simulink model "plots"  (R2014b)
settings: Solver=FixedStepDiscrete  StartTime=0.0  StopTime=inf  FixedStep=Ts  RelTol=1e-3
InitFcn:
  | Ts=0.010;
  | ROBOT_DOF=23;
  | robotName='icubGazeboSim';
  | localName='simulink';
libraries: WBCLibrary x2
settings Model: Creator=jorhabib  LastModifiedBy=jorhabib

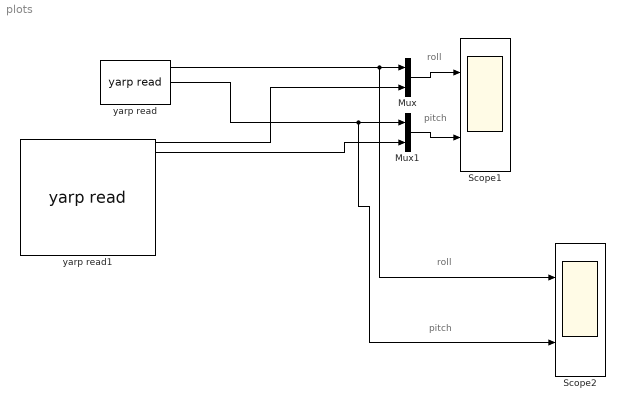
== system plots ==
  note: pitch
  note: roll
  note: roll
  note: pitch
  Mux : Mux  Inputs=2
  Mux1 : Mux  Inputs=2
  Scope1 : Scope  NumInputPorts=2
      settings: TimeRange=50000  YMin=-50~-60  YMax=40~60
  Scope2 : Scope  NumInputPorts=2
      settings: TimeRange=50000  YMin=0~0  YMax=1~1  SaveName=ScopeData2
  yarp read : WBCLibrary/Utilities/yarp read  from=['/' 'quaternionEKFModule' '/filteredOrientationEuler:o']  to='...'  num=3  blocking=off  timestamp=off  autoconnect=on
  yarp read1 : WBCLibrary/Utilities/yarp read  from=['/icub/inertial']  to='...'  num=12  blocking=off  timestamp=off  autoconnect=on
  wires:
  yarp read/1 -> Scope2/1, Mux/1
  yarp read1/1 -> Mux/2
  yarp read/2 -> Scope2/2, Mux1/1
  yarp read1/2 -> Mux1/2
  Mux/1 -> Scope1/1
  Mux1/1 -> Scope1/2
